simulink model "amplifierboard"  (R2020b)
settings: Solver=FixedStepDiscrete  StartTime=0.0  StopTime=2  FixedStep=0.01  RelTol=1e-3
InitFcn:
  | mbd_s32k_consistency_checks(bdroot(gcs));
undefined symbols (not defined in the file): AutoLowerVal, AutoRaiseVal, HoldVal, LED_En, LED_Off, LED_On, Logic_High, Logic_Low, LQFP, ManualLowerVal, ManualRaiseVal, PWRWNDW_CHDLCK, sC_bool_PWMEN, sC_cnt_FWSetting, sC_cnt_Mtr_DrvNo_HB, sC_cnt_PWMHB1to4, sC_cnt_PWMHB5to8, sC_cnt_TargetSlowRange, sC_pct_ManualMax, sC_pct_RampDwn, sC_pct_RampUp, sC_pct_StartPWM, sC_pct_Targetmax, SwitchPackRangeOffset, Threshold_Value, Tolerant_Time
libraries: mbd_s32k1xx_ec_toolbox x205, simulink x59, canmsglib x19, Filter x15, wndwcmd x3
(part 4 of 6)

== system amplifierboard/CAN_Receive_And_Unpack/Subsystem/Chart/SendPos31StopPosResp ==
  f : TriggerPort  TriggerType=function-call  VariantControl=(inherit)
      settings: CopyFcn=Stateflow.SLINSF.SimulinkMan.removeBlockPreDeleteFcn  PreDeleteFcn=Stateflow.SLINSF.SimulinkMan.unsafePredeleteFcn
  FCAN_Send_ID_0xAA : mbd_s32k1xx_ec_toolbox/Communication Blocks/CAN Blocks/FCAN_Send  Priority=2  can_instance=1  can_mode=Non-blocking  can_timeout_ms=0  can_mb_idx=29  can_mb_init=On each call  show_id_input=off  can_extended_id=off  can_is_remote=off  can_id=AA  show_adv_opts=on  can_fd_enable=off  can_enable_brs=on  can_fd_padding=0
  Generate_Data : Subsystem
  wires:
  Generate_Data/2(Length) -> FCAN_Send_ID_0xAA/2
  Generate_Data/1(Data) -> FCAN_Send_ID_0xAA/1

== system amplifierboard/CAN_Receive_And_Unpack/Subsystem/If Action Subsystem1 ==
  TImeStamp : Inport
  Action Port : ActionPort  ActionPortLabel=if((u1 ~= u2) | ( u3 == 1))
  Constant : Constant  OutDataTypeStr=boolean
  Data Store Write : DataStoreWrite  DataStoreName=PreviousTimeStamp
  Data Store Write1 : DataStoreWrite  DataStoreName=NewMsgRXed
  wires:
  TImeStamp/1 -> Data Store Write/1
  Constant/1 -> Data Store Write1/1

== system amplifierboard/CAN_Receive_And_Unpack/Subsystem/If Action Subsystem2 ==
  Action Port : ActionPort  ActionPortLabel=else
  Constant : Constant  Value=0  OutDataTypeStr=boolean
  Data Store Write1 : DataStoreWrite  DataStoreName=NewMsgRXed
  wires:
  Constant/1 -> Data Store Write1/1

== system amplifierboard/CAN_Receive_And_Unpack/Subsystem1/Fold_Unfold ==
  Input : Inport
  Input1 : Inport  Port=2
  Compare To Constant : simulink/Logic and Bit Operations/Compare To Constant  relop===  const=1.0  OutDataTypeStr=boolean
  Compare To Constant{1..2,4..5} (4 alike) : simulink/Logic and Bit Operations/Compare To Constant  relop===  const=0  OutDataTypeStr=boolean
  Compare To Constant3 : simulink/Logic and Bit Operations/Compare To Constant  relop===  const=1  OutDataTypeStr=boolean
  Compare To Constant6 : simulink/Logic and Bit Operations/Compare To Constant  relop===  const=1  OutDataTypeStr=boolean
  Compare To Constant7 : simulink/Logic and Bit Operations/Compare To Constant  relop===  const=1  OutDataTypeStr=boolean
  If : If  NumInputs=4  IfExpression=u1 == 1  ElseIfExpressions=u2 == 1, u3 == 1 , u4 == 1  ShowElse=off
  If Action Subsystem : Subsystem  TreatAsAtomicUnit=on
  If Action Subsystem1 : Subsystem  TreatAsAtomicUnit=on
  If Action Subsystem2 : Subsystem  TreatAsAtomicUnit=on
  If Action Subsystem3 : Subsystem  TreatAsAtomicUnit=on
  Logical Operator{,1..3} (4 alike) : Logic  AllPortsSameDT=off  OutDataTypeStr=boolean
  Merge : Merge  Inputs=4
  Motor : Outport
  wires:
  Input1/1 -> Compare To Constant7/1, Compare To Constant5/1, Compare To Constant3/1, Compare To Constant1/1
  Compare To Constant5/1 -> Logical Operator2/2
  If Action Subsystem/1("Forward_Direction ") -> Merge/1
  If/2 -> If Action Subsystem1/Action
  Compare To Constant2/1 -> Logical Operator1/1
  Compare To Constant4/1 -> Logical Operator2/1
  Compare To Constant3/1 -> Logical Operator1/2
  Compare To Constant/1 -> Logical Operator/1
  Logical Operator3/1 -> If/4
  Input/1 -> Compare To Constant2/1, Compare To Constant4/1, Compare To Constant6/1, Compare To Constant/1
  Compare To Constant7/1 -> Logical Operator3/2
  If/4 -> If Action Subsystem3/Action
  Compare To Constant6/1 -> Logical Operator3/1
  Merge/1 -> Motor/1
  If Action Subsystem1/1(Reverse_Direction) -> Merge/2
  If Action Subsystem3/1(Standstill_invalid) -> Merge/4
  If Action Subsystem2/1(Standstill_Invalid) -> Merge/3
  If/1 -> If Action Subsystem/Action
  Logical Operator2/1 -> If/3
  Logical Operator1/1 -> If/2
  Compare To Constant1/1 -> Logical Operator/2
  If/3 -> If Action Subsystem2/Action
  Logical Operator/1 -> If/1

== system amplifierboard/CAN_Receive_And_Unpack/Subsystem1/LED1DR_PWM ==
  In1 : Inport
  Data Type Conversion1 : DataTypeConversion  OutDataTypeStr=Enum: LED_En
  Data Type Conversion11 : DataTypeConversion  OutDataTypeStr=Enum: LED_En
  Digital_Output : mbd_s32k1xx_ec_toolbox/GPIO Blocks/Digital_Output  gpio_pin=PTD8: [PTD8 | Port D I/O]  init_val=Low  drive_strength=High
  Enumerated Constant1 : simulink/Sources/Enumerated Constant  OutDataTypeStr=Enum: LED_En  Value=LED_En.DISABLE  SampleTime=inf
  Enumerated Constant6 : simulink/Sources/Enumerated Constant  OutDataTypeStr=Enum: LED_En  Value=LED_En.ENABLE  SampleTime=inf
  LED_Off : Constant  Value=LED_Off  OutDataTypeStr=Inherit: Inherit via back propagation
  LED_On : Constant  Value=LED_On  OutDataTypeStr=Inherit: Inherit via back propagation
  Relational Operator1 : RelationalOperator  Operator===  OutDataTypeStr=boolean  RndMeth=Simplest
  Relational Operator6 : RelationalOperator  Operator===  OutDataTypeStr=boolean  RndMeth=Simplest
  Switch : Switch  Criteria=u2 > Threshold
  Switch1 : Switch  Criteria=u2 > Threshold
  Unit Delay : UnitDelay  SampleTime=-1  HasFrameUpgradeWarning=on
  wires:
  In1/1 -> Data Type Conversion11/1, Data Type Conversion1/1
  Switch1/1 -> Switch/3
  LED_Off/1 -> Switch1/1
  Enumerated Constant6/1 -> Relational Operator6/2
  Data Type Conversion11/1 -> Relational Operator6/1
  Relational Operator1/1 -> Switch1/2
  Relational Operator6/1 -> Switch/2
  LED_On/1 -> Switch/1
  Switch/1 -> Unit Delay/1, Digital_Output/1
  Enumerated Constant1/1 -> Relational Operator1/2
  Data Type Conversion1/1 -> Relational Operator1/1
  Unit Delay/1 -> Switch1/3

== system amplifierboard/CAN_Receive_And_Unpack/Subsystem1/LED2DR_PWM ==
  In1 : Inport
  Data Type Conversion1 : DataTypeConversion  OutDataTypeStr=Enum: LED_En
  Data Type Conversion11 : DataTypeConversion  OutDataTypeStr=Enum: LED_En
  Digital_Output : mbd_s32k1xx_ec_toolbox/GPIO Blocks/Digital_Output  gpio_pin=PTD9: [PTD9 | Port D I/O]  init_val=Low  drive_strength=High
  Enumerated Constant1 : simulink/Sources/Enumerated Constant  OutDataTypeStr=Enum: LED_En  Value=LED_En.DISABLE  SampleTime=inf
  Enumerated Constant6 : simulink/Sources/Enumerated Constant  OutDataTypeStr=Enum: LED_En  Value=LED_En.ENABLE  SampleTime=inf
  LED_Off : Constant  Value=LED_Off  OutDataTypeStr=Inherit: Inherit via back propagation
  LED_On : Constant  Value=LED_On  OutDataTypeStr=Inherit: Inherit via back propagation
  Relational Operator1 : RelationalOperator  Operator===  OutDataTypeStr=boolean  RndMeth=Simplest
  Relational Operator6 : RelationalOperator  Operator===  OutDataTypeStr=boolean  RndMeth=Simplest
  Switch : Switch  Criteria=u2 > Threshold
  Switch1 : Switch  Criteria=u2 > Threshold
  Unit Delay : UnitDelay  SampleTime=-1  HasFrameUpgradeWarning=on
  wires:
  Unit Delay/1 -> Switch1/3
  Data Type Conversion1/1 -> Relational Operator1/1
  Enumerated Constant1/1 -> Relational Operator1/2
  Switch/1 -> Digital_Output/1, Unit Delay/1
  LED_On/1 -> Switch/1
  Relational Operator6/1 -> Switch/2
  Relational Operator1/1 -> Switch1/2
  Data Type Conversion11/1 -> Relational Operator6/1
  Enumerated Constant6/1 -> Relational Operator6/2
  LED_Off/1 -> Switch1/1
  Switch1/1 -> Switch/3
  In1/1 -> Data Type Conversion1/1, Data Type Conversion11/1

== system amplifierboard/CAN_Receive_And_Unpack/Subsystem1/LED3DR_PWM ==
  In1 : Inport
  Data Type Conversion1 : DataTypeConversion  OutDataTypeStr=Enum: LED_En
  Data Type Conversion11 : DataTypeConversion  OutDataTypeStr=Enum: LED_En
  Digital_Output : mbd_s32k1xx_ec_toolbox/GPIO Blocks/Digital_Output  gpio_pin=PTC13: [PTC13 | Port C I/O]  init_val=Low  drive_strength=High
  Enumerated Constant1 : simulink/Sources/Enumerated Constant  OutDataTypeStr=Enum: LED_En  Value=LED_En.DISABLE  SampleTime=inf
  Enumerated Constant6 : simulink/Sources/Enumerated Constant  OutDataTypeStr=Enum: LED_En  Value=LED_En.ENABLE  SampleTime=inf
  LED_Off : Constant  Value=LED_Off  OutDataTypeStr=Inherit: Inherit via back propagation
  LED_On : Constant  Value=LED_On  OutDataTypeStr=Inherit: Inherit via back propagation
  Relational Operator1 : RelationalOperator  Operator===  OutDataTypeStr=boolean  RndMeth=Simplest
  Relational Operator6 : RelationalOperator  Operator===  OutDataTypeStr=boolean  RndMeth=Simplest
  Switch : Switch  Criteria=u2 > Threshold
  Switch1 : Switch  Criteria=u2 > Threshold
  Unit Delay : UnitDelay  SampleTime=-1  HasFrameUpgradeWarning=on
  wires:
  In1/1 -> Data Type Conversion11/1, Data Type Conversion1/1
  Switch1/1 -> Switch/3
  LED_Off/1 -> Switch1/1
  Enumerated Constant6/1 -> Relational Operator6/2
  Data Type Conversion11/1 -> Relational Operator6/1
  Relational Operator1/1 -> Switch1/2
  Relational Operator6/1 -> Switch/2
  LED_On/1 -> Switch/1
  Switch/1 -> Unit Delay/1, Digital_Output/1
  Enumerated Constant1/1 -> Relational Operator1/2
  Data Type Conversion1/1 -> Relational Operator1/1
  Unit Delay/1 -> Switch1/3

== system amplifierboard/CAN_Receive_And_Unpack/Subsystem1/LED4DR_PWM ==
  In1 : Inport
  Data Type Conversion1 : DataTypeConversion  OutDataTypeStr=Enum: LED_En
  Data Type Conversion11 : DataTypeConversion  OutDataTypeStr=Enum: LED_En
  Digital_Output : mbd_s32k1xx_ec_toolbox/GPIO Blocks/Digital_Output  gpio_pin=PTC10: [PTC10 | Port C I/O]  init_val=Low  drive_strength=High
  Enumerated Constant1 : simulink/Sources/Enumerated Constant  OutDataTypeStr=Enum: LED_En  Value=LED_En.DISABLE  SampleTime=inf
  Enumerated Constant6 : simulink/Sources/Enumerated Constant  OutDataTypeStr=Enum: LED_En  Value=LED_En.ENABLE  SampleTime=inf
  LED_Off : Constant  Value=LED_Off  OutDataTypeStr=Inherit: Inherit via back propagation
  LED_On : Constant  Value=LED_On  OutDataTypeStr=Inherit: Inherit via back propagation
  Relational Operator1 : RelationalOperator  Operator===  OutDataTypeStr=boolean  RndMeth=Simplest
  Relational Operator6 : RelationalOperator  Operator===  OutDataTypeStr=boolean  RndMeth=Simplest
  Switch : Switch  Criteria=u2 > Threshold
  Switch1 : Switch  Criteria=u2 > Threshold
  Unit Delay : UnitDelay  SampleTime=-1  HasFrameUpgradeWarning=on
  wires:
  Unit Delay/1 -> Switch1/3
  Data Type Conversion1/1 -> Relational Operator1/1
  Enumerated Constant1/1 -> Relational Operator1/2
  Switch/1 -> Digital_Output/1, Unit Delay/1
  LED_On/1 -> Switch/1
  Relational Operator6/1 -> Switch/2
  Relational Operator1/1 -> Switch1/2
  Data Type Conversion11/1 -> Relational Operator6/1
  Enumerated Constant6/1 -> Relational Operator6/2
  LED_Off/1 -> Switch1/1
  Switch1/1 -> Switch/3
  In1/1 -> Data Type Conversion1/1, Data Type Conversion11/1

== system amplifierboard/CAN_Receive_And_Unpack/Subsystem1/LED5DR_PWM ==
  In1 : Inport
  Data Type Conversion1 : DataTypeConversion  OutDataTypeStr=Enum: LED_En
  Data Type Conversion11 : DataTypeConversion  OutDataTypeStr=Enum: LED_En
  Digital_Output : mbd_s32k1xx_ec_toolbox/GPIO Blocks/Digital_Output  gpio_pin=PTC11: [PTC11 | Port C I/O]  init_val=Low  drive_strength=High
  Enumerated Constant1 : simulink/Sources/Enumerated Constant  OutDataTypeStr=Enum: LED_En  Value=LED_En.DISABLE  SampleTime=inf
  Enumerated Constant6 : simulink/Sources/Enumerated Constant  OutDataTypeStr=Enum: LED_En  Value=LED_En.ENABLE  SampleTime=inf
  LED_Off : Constant  Value=LED_Off  OutDataTypeStr=Inherit: Inherit via back propagation
  LED_On : Constant  Value=LED_On  OutDataTypeStr=Inherit: Inherit via back propagation
  Relational Operator1 : RelationalOperator  Operator===  OutDataTypeStr=boolean  RndMeth=Simplest
  Relational Operator6 : RelationalOperator  Operator===  OutDataTypeStr=boolean  RndMeth=Simplest
  Switch : Switch  Criteria=u2 > Threshold
  Switch1 : Switch  Criteria=u2 > Threshold
  Unit Delay : UnitDelay  SampleTime=-1  HasFrameUpgradeWarning=on
  wires:
  In1/1 -> Data Type Conversion11/1, Data Type Conversion1/1
  Switch1/1 -> Switch/3
  LED_Off/1 -> Switch1/1
  Enumerated Constant6/1 -> Relational Operator6/2
  Data Type Conversion11/1 -> Relational Operator6/1
  Relational Operator1/1 -> Switch1/2
  Relational Operator6/1 -> Switch/2
  LED_On/1 -> Switch/1
  Switch/1 -> Unit Delay/1, Digital_Output/1
  Enumerated Constant1/1 -> Relational Operator1/2
  Data Type Conversion1/1 -> Relational Operator1/1
  Unit Delay/1 -> Switch1/3

== system amplifierboard/CAN_Receive_And_Unpack/Subsystem1/LED6DR_PWM ==
  In1 : Inport
  Data Type Conversion1 : DataTypeConversion  OutDataTypeStr=Enum: LED_En
  Data Type Conversion11 : DataTypeConversion  OutDataTypeStr=Enum: LED_En
  Digital_Output : mbd_s32k1xx_ec_toolbox/GPIO Blocks/Digital_Output  gpio_pin=PTC9: [PTC9 | Port C I/O]  init_val=Low  drive_strength=High
  Enumerated Constant1 : simulink/Sources/Enumerated Constant  OutDataTypeStr=Enum: LED_En  Value=LED_En.DISABLE  SampleTime=inf
  Enumerated Constant6 : simulink/Sources/Enumerated Constant  OutDataTypeStr=Enum: LED_En  Value=LED_En.ENABLE  SampleTime=inf
  LED_Off : Constant  Value=LED_Off  OutDataTypeStr=Inherit: Inherit via back propagation
  LED_On : Constant  Value=LED_On  OutDataTypeStr=Inherit: Inherit via back propagation
  Relational Operator1 : RelationalOperator  Operator===  OutDataTypeStr=boolean  RndMeth=Simplest
  Relational Operator6 : RelationalOperator  Operator===  OutDataTypeStr=boolean  RndMeth=Simplest
  Switch : Switch  Criteria=u2 > Threshold
  Switch1 : Switch  Criteria=u2 > Threshold
  Unit Delay : UnitDelay  SampleTime=-1  HasFrameUpgradeWarning=on
  wires:
  Unit Delay/1 -> Switch1/3
  Data Type Conversion1/1 -> Relational Operator1/1
  Enumerated Constant1/1 -> Relational Operator1/2
  Switch/1 -> Digital_Output/1, Unit Delay/1
  LED_On/1 -> Switch/1
  Relational Operator6/1 -> Switch/2
  Relational Operator1/1 -> Switch1/2
  Data Type Conversion11/1 -> Relational Operator6/1
  Enumerated Constant6/1 -> Relational Operator6/2
  LED_Off/1 -> Switch1/1
  Switch1/1 -> Switch/3
  In1/1 -> Data Type Conversion1/1, Data Type Conversion11/1

== system amplifierboard/CAN_Receive_And_Unpack/Subsystem1/Motor4 ==
  Input : Inport
  Input1 : Inport  Port=2
  Compare To Constant : simulink/Logic and Bit Operations/Compare To Constant  relop===  const=1.0  OutDataTypeStr=boolean
  Compare To Constant{1..2,4..5} (4 alike) : simulink/Logic and Bit Operations/Compare To Constant  relop===  const=0  OutDataTypeStr=boolean
  Compare To Constant3 : simulink/Logic and Bit Operations/Compare To Constant  relop===  const=1  OutDataTypeStr=boolean
  Compare To Constant6 : simulink/Logic and Bit Operations/Compare To Constant  relop===  const=1  OutDataTypeStr=boolean
  Compare To Constant7 : simulink/Logic and Bit Operations/Compare To Constant  relop===  const=1  OutDataTypeStr=boolean
  If : If  NumInputs=4  IfExpression=u1 == 1  ElseIfExpressions=u2 == 1, u3 == 1 , u4 == 1  ShowElse=off
  If Action Subsystem : Subsystem  TreatAsAtomicUnit=on
  If Action Subsystem1 : Subsystem  TreatAsAtomicUnit=on
  If Action Subsystem2 : Subsystem  TreatAsAtomicUnit=on
  If Action Subsystem3 : Subsystem  TreatAsAtomicUnit=on
  Logical Operator{,1..3} (4 alike) : Logic  AllPortsSameDT=off  OutDataTypeStr=boolean
  Merge : Merge  Inputs=4
  Motor : Outport
  wires:
  Logical Operator/1 -> If/1
  If/3 -> If Action Subsystem2/Action
  Compare To Constant1/1 -> Logical Operator/2
  Logical Operator1/1 -> If/2
  Logical Operator2/1 -> If/3
  If/1 -> If Action Subsystem/Action
  If Action Subsystem2/1(Standstill_Invalid) -> Merge/3
  If Action Subsystem3/1(Standstill_invalid) -> Merge/4
  If Action Subsystem1/1(Reverse_Direction) -> Merge/2
  Merge/1 -> Motor/1
  Compare To Constant6/1 -> Logical Operator3/1
  If/4 -> If Action Subsystem3/Action
  Compare To Constant7/1 -> Logical Operator3/2
  Input/1 -> Compare To Constant/1, Compare To Constant6/1, Compare To Constant4/1, Compare To Constant2/1
  Logical Operator3/1 -> If/4
  Compare To Constant/1 -> Logical Operator/1
  Compare To Constant3/1 -> Logical Operator1/2
  Compare To Constant4/1 -> Logical Operator2/1
  Compare To Constant2/1 -> Logical Operator1/1
  If/2 -> If Action Subsystem1/Action
  If Action Subsystem/1("Forward_Direction ") -> Merge/1
  Compare To Constant5/1 -> Logical Operator2/2
  Input1/1 -> Compare To Constant1/1, Compare To Constant3/1, Compare To Constant5/1, Compare To Constant7/1

== system amplifierboard/CAN_Receive_And_Unpack/Subsystem1/Motor5 ==
  Input : Inport
  Heating : Inport  Port=2
  Compare To Constant : simulink/Logic and Bit Operations/Compare To Constant  relop===  const=1.0  OutDataTypeStr=boolean
  Compare To Constant1 : simulink/Logic and Bit Operations/Compare To Constant  relop===  const=0  OutDataTypeStr=boolean
  Compare To Constant2 : simulink/Logic and Bit Operations/Compare To Constant  relop===  const=0  OutDataTypeStr=boolean
  Compare To Constant3 : simulink/Logic and Bit Operations/Compare To Constant  relop===  const=1  OutDataTypeStr=boolean
  If : If  NumInputs=2  IfExpression=u2 == 1
  If Action Subsystem : Subsystem  TreatAsAtomicUnit=on
  If Action Subsystem1 : Subsystem  TreatAsAtomicUnit=on
  Logical Operator : Logic  AllPortsSameDT=off  OutDataTypeStr=boolean
  Logical Operator1 : Logic  AllPortsSameDT=off  OutDataTypeStr=boolean
  Merge : Merge
  Motor : Outport
  wires:
  Heating/1 -> Compare To Constant1/1, Compare To Constant3/1
  If Action Subsystem/1("Forward_Direction ") -> Merge/1
  If/2 -> If Action Subsystem1/Action
  Compare To Constant2/1 -> Logical Operator1/1
  Compare To Constant3/1 -> Logical Operator1/2
  Compare To Constant/1 -> Logical Operator/1
  Input/1 -> Compare To Constant2/1, Compare To Constant/1
  Merge/1 -> Motor/1
  If Action Subsystem1/1(Standstill_Invalid) -> Merge/2
  If/1 -> If Action Subsystem/Action
  Logical Operator1/1 -> If/2
  Compare To Constant1/1 -> Logical Operator/2
  Logical Operator/1 -> If/1

== system amplifierboard/CAN_Receive_And_Unpack/Subsystem1/Motor6 ==
  Input : Inport
  Input1 : Inport  Port=2
  Compare To Constant : simulink/Logic and Bit Operations/Compare To Constant  relop===  const=1.0  OutDataTypeStr=boolean
  Compare To Constant{1..2,4..5} (4 alike) : simulink/Logic and Bit Operations/Compare To Constant  relop===  const=0  OutDataTypeStr=boolean
  Compare To Constant3 : simulink/Logic and Bit Operations/Compare To Constant  relop===  const=1  OutDataTypeStr=boolean
  Compare To Constant6 : simulink/Logic and Bit Operations/Compare To Constant  relop===  const=1  OutDataTypeStr=boolean
  Compare To Constant7 : simulink/Logic and Bit Operations/Compare To Constant  relop===  const=1  OutDataTypeStr=boolean
  If : If  NumInputs=4  IfExpression=u1 == 1  ElseIfExpressions=u2 == 1, u3 == 1 , u4 == 1  ShowElse=off
  If Action Subsystem : Subsystem  TreatAsAtomicUnit=on
  If Action Subsystem1 : Subsystem  TreatAsAtomicUnit=on
  If Action Subsystem2 : Subsystem  TreatAsAtomicUnit=on
  If Action Subsystem3 : Subsystem  TreatAsAtomicUnit=on
  Logical Operator{,1..3} (4 alike) : Logic  AllPortsSameDT=off  OutDataTypeStr=boolean
  Merge : Merge  Inputs=4
  Motor : Outport
  wires:
  Logical Operator/1 -> If/1
  If/3 -> If Action Subsystem2/Action
  Compare To Constant1/1 -> Logical Operator/2
  Logical Operator1/1 -> If/2
  Logical Operator2/1 -> If/3
  If/1 -> If Action Subsystem/Action
  If Action Subsystem2/1(Standstill_Invalid) -> Merge/3
  If Action Subsystem3/1(Standstill_invalid) -> Merge/4
  If Action Subsystem1/1(Reverse_Direction) -> Merge/2
  Merge/1 -> Motor/1
  Compare To Constant6/1 -> Logical Operator3/1
  If/4 -> If Action Subsystem3/Action
  Compare To Constant7/1 -> Logical Operator3/2
  Input/1 -> Compare To Constant/1, Compare To Constant6/1, Compare To Constant4/1, Compare To Constant2/1
  Logical Operator3/1 -> If/4
  Compare To Constant/1 -> Logical Operator/1
  Compare To Constant3/1 -> Logical Operator1/2
  Compare To Constant4/1 -> Logical Operator2/1
  Compare To Constant2/1 -> Logical Operator1/1
  If/2 -> If Action Subsystem1/Action
  If Action Subsystem/1("Forward_Direction ") -> Merge/1
  Compare To Constant5/1 -> Logical Operator2/2
  Input1/1 -> Compare To Constant1/1, Compare To Constant3/1, Compare To Constant5/1, Compare To Constant7/1

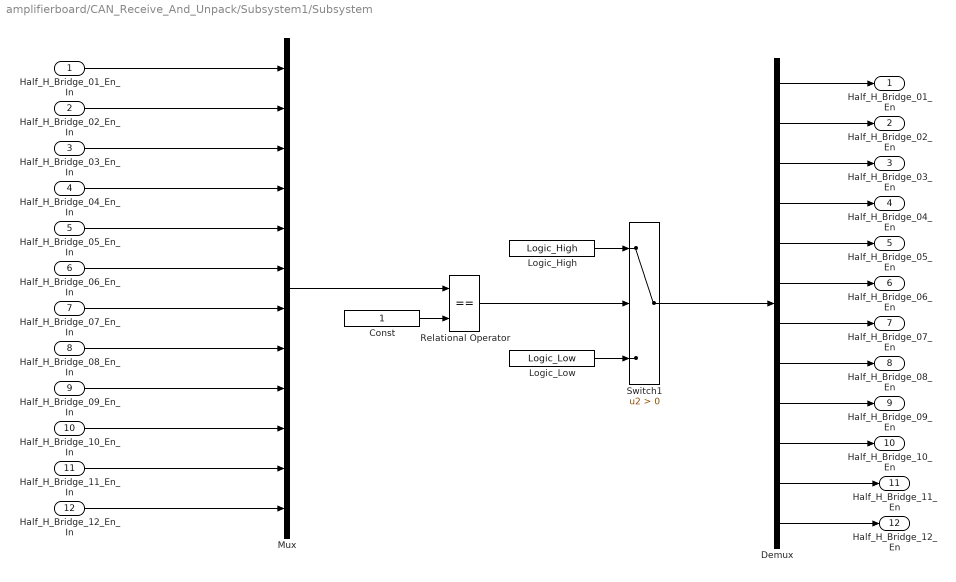
== system amplifierboard/CAN_Receive_And_Unpack/Subsystem1/Subsystem ==
  Half_H_Bridge_01_En_In : Inport
  Half_H_Bridge_02_En_In : Inport  Port=2
  Half_H_Bridge_03_En_In : Inport  Port=3
  Half_H_Bridge_04_En_In : Inport  Port=4
  Half_H_Bridge_05_En_In : Inport  Port=5
  Half_H_Bridge_06_En_In : Inport  Port=6
  Half_H_Bridge_07_En_In : Inport  Port=7
  Half_H_Bridge_08_En_In : Inport  Port=8
  Half_H_Bridge_09_En_In : Inport  Port=9
  Half_H_Bridge_10_En_In : Inport  Port=10
  Half_H_Bridge_11_En_In : Inport  Port=11
  Half_H_Bridge_12_En_In : Inport  Port=12
  Const : Constant  OutDataTypeStr=Inherit: Inherit via back propagation
  Demux : Demux  Outputs=12
  Logic_High : Constant  Value=Logic_High  OutDataTypeStr=Inherit: Inherit via back propagation
  Logic_Low : Constant  Value=Logic_Low  OutDataTypeStr=Inherit: Inherit via back propagation
  Mux : Mux  Inputs=12
  Relational Operator : RelationalOperator  Operator===  OutDataTypeStr=boolean  RndMeth=Simplest
  Switch1 : Switch  Criteria=u2 > Threshold
  Half_H_Bridge_01_En : Outport
  Half_H_Bridge_02_En : Outport  Port=2
  Half_H_Bridge_03_En : Outport  Port=3
  Half_H_Bridge_04_En : Outport  Port=4
  Half_H_Bridge_05_En : Outport  Port=5
  Half_H_Bridge_06_En : Outport  Port=6
  Half_H_Bridge_07_En : Outport  Port=7
  Half_H_Bridge_08_En : Outport  Port=8
  Half_H_Bridge_09_En : Outport  Port=9
  Half_H_Bridge_10_En : Outport  Port=10
  Half_H_Bridge_11_En : Outport  Port=11
  Half_H_Bridge_12_En : Outport  Port=12
  wires:
  Relational Operator/1 -> Switch1/2
  Switch1/1 -> Demux/1
  Demux/1 -> Half_H_Bridge_01_En/1
  Half_H_Bridge_02_En_In/1 -> Mux/2
  Half_H_Bridge_03_En_In/1 -> Mux/3
  Half_H_Bridge_04_En_In/1 -> Mux/4
  Half_H_Bridge_05_En_In/1 -> Mux/5
  Demux/2 -> Half_H_Bridge_02_En/1
  Demux/3 -> Half_H_Bridge_03_En/1
  Demux/4 -> Half_H_Bridge_04_En/1
  Demux/5 -> Half_H_Bridge_05_En/1
  Half_H_Bridge_06_En_In/1 -> Mux/6
  Half_H_Bridge_07_En_In/1 -> Mux/7
  Half_H_Bridge_08_En_In/1 -> Mux/8
  Half_H_Bridge_09_En_In/1 -> Mux/9
  Half_H_Bridge_10_En_In/1 -> Mux/10
  Half_H_Bridge_11_En_In/1 -> Mux/11
  Half_H_Bridge_12_En_In/1 -> Mux/12
  Demux/6 -> Half_H_Bridge_06_En/1
  Demux/7 -> Half_H_Bridge_07_En/1
  Demux/8 -> Half_H_Bridge_08_En/1
  Demux/9 -> Half_H_Bridge_09_En/1
  Demux/10 -> Half_H_Bridge_10_En/1
  Demux/11 -> Half_H_Bridge_11_En/1
  Demux/12 -> Half_H_Bridge_12_En/1
  Half_H_Bridge_01_En_In/1 -> Mux/1
  Mux/1 -> Relational Operator/1
  Const/1 -> Relational Operator/2
  Logic_Low/1 -> Switch1/3
  Logic_High/1 -> Switch1/1

== system amplifierboard/CAN_Receive_And_Unpack/Subsystem1/Subsystem1 ==
  mirror_common : Inport
  right_left : Inport  Port=2
  up_down : Inport  Port=3
  Motor2 : Subsystem
  Motor3 : Subsystem
  Motor4 : Outport
  Motor5 : Outport  Port=2
  wires:
  Motor2/1(Motor) -> Motor4/1
  Motor3/1(Motor) -> Motor5/1
  up_down/1 -> Motor3/1(Input)
  right_left/1 -> Motor2/1(Input)
  mirror_common/1 -> Motor3/2(Input1), Motor2/2(Input1)

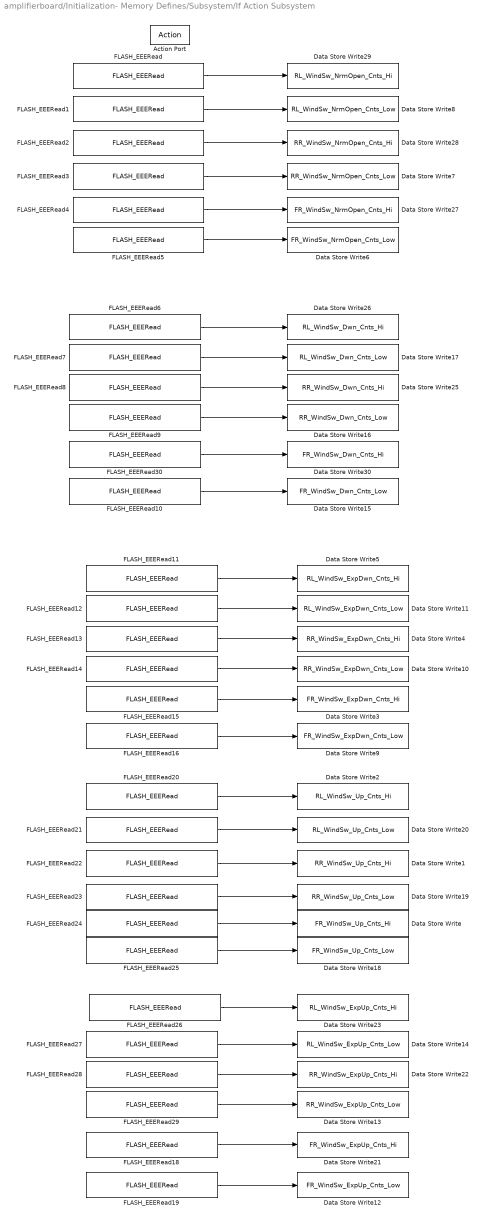
== system amplifierboard/Initialization- Memory Defines/Subsystem/If Action Subsystem ==
  Action Port : ActionPort  ActionPortLabel=if((u1 <= 1200) & (u2 <= 750))
  Data Store Write : DataStoreWrite  DataStoreName=FR_WindSw_Up_Cnts_Hi
  Data Store Write1 : DataStoreWrite  DataStoreName=RR_WindSw_Up_Cnts_Hi
  Data Store Write10 : DataStoreWrite  DataStoreName=RR_WindSw_ExpDwn_Cnts_Low
  Data Store Write11 : DataStoreWrite  DataStoreName=RL_WindSw_ExpDwn_Cnts_Low
  Data Store Write12 : DataStoreWrite  DataStoreName=FR_WindSw_ExpUp_Cnts_Low
  Data Store Write13 : DataStoreWrite  DataStoreName=RR_WindSw_ExpUp_Cnts_Low
  Data Store Write14 : DataStoreWrite  DataStoreName=RL_WindSw_ExpUp_Cnts_Low
  Data Store Write15 : DataStoreWrite  DataStoreName=FR_WindSw_Dwn_Cnts_Low
  Data Store Write16 : DataStoreWrite  DataStoreName=RR_WindSw_Dwn_Cnts_Low
  Data Store Write17 : DataStoreWrite  DataStoreName=RL_WindSw_Dwn_Cnts_Low
  Data Store Write18 : DataStoreWrite  DataStoreName=FR_WindSw_Up_Cnts_Low
  Data Store Write19 : DataStoreWrite  DataStoreName=RR_WindSw_Up_Cnts_Low
  Data Store Write2 : DataStoreWrite  DataStoreName=RL_WindSw_Up_Cnts_Hi
  Data Store Write20 : DataStoreWrite  DataStoreName=RL_WindSw_Up_Cnts_Low
  Data Store Write21 : DataStoreWrite  DataStoreName=FR_WindSw_ExpUp_Cnts_Hi
  Data Store Write22 : DataStoreWrite  DataStoreName=RR_WindSw_ExpUp_Cnts_Hi
  Data Store Write23 : DataStoreWrite  DataStoreName=RL_WindSw_ExpUp_Cnts_Hi
  Data Store Write25 : DataStoreWrite  DataStoreName=RR_WindSw_Dwn_Cnts_Hi
  Data Store Write26 : DataStoreWrite  DataStoreName=RL_WindSw_Dwn_Cnts_Hi
  Data Store Write27 : DataStoreWrite  DataStoreName=FR_WindSw_NrmOpen_Cnts_Hi
  Data Store Write28 : DataStoreWrite  DataStoreName=RR_WindSw_NrmOpen_Cnts_Hi
  Data Store Write29 : DataStoreWrite  DataStoreName=RL_WindSw_NrmOpen_Cnts_Hi
  Data Store Write3 : DataStoreWrite  DataStoreName=FR_WindSw_ExpDwn_Cnts_Hi
  Data Store Write30 : DataStoreWrite  DataStoreName=FR_WindSw_Dwn_Cnts_Hi
  Data Store Write4 : DataStoreWrite  DataStoreName=RR_WindSw_ExpDwn_Cnts_Hi
  Data Store Write5 : DataStoreWrite  DataStoreName=RL_WindSw_ExpDwn_Cnts_Hi
  Data Store Write6 : DataStoreWrite  DataStoreName=FR_WindSw_NrmOpen_Cnts_Low
  Data Store Write7 : DataStoreWrite  DataStoreName=RR_WindSw_NrmOpen_Cnts_Low
  Data Store Write8 : DataStoreWrite  DataStoreName=RL_WindSw_NrmOpen_Cnts_Low
  Data Store Write9 : DataStoreWrite  DataStoreName=FR_WindSw_ExpDwn_Cnts_Low
  FLASH_EEERead : mbd_s32k1xx_ec_toolbox/Core and System Blocks/FLASH Blocks/FLASH_EEERead  base=0x14000000  offset=0x0F00  ptr=uint16_t
  FLASH_EEERead1 : mbd_s32k1xx_ec_toolbox/Core and System Blocks/FLASH Blocks/FLASH_EEERead  base=0x14000000  offset=0x0F02  ptr=uint16_t
  FLASH_EEERead10 : mbd_s32k1xx_ec_toolbox/Core and System Blocks/FLASH Blocks/FLASH_EEERead  base=0x14000000  offset=0x0F16  ptr=uint16_t
  FLASH_EEERead11 : mbd_s32k1xx_ec_toolbox/Core and System Blocks/FLASH Blocks/FLASH_EEERead  base=0x14000000  offset=0x0F18  ptr=uint16_t
  FLASH_EEERead12 : mbd_s32k1xx_ec_toolbox/Core and System Blocks/FLASH Blocks/FLASH_EEERead  base=0x14000000  offset=0x0F1A  ptr=uint16_t
  FLASH_EEERead13 : mbd_s32k1xx_ec_toolbox/Core and System Blocks/FLASH Blocks/FLASH_EEERead  base=0x14000000  offset=0x0F1C  ptr=uint16_t
  FLASH_EEERead14 : mbd_s32k1xx_ec_toolbox/Core and System Blocks/FLASH Blocks/FLASH_EEERead  base=0x14000000  offset=0x0F1E  ptr=uint16_t
  FLASH_EEERead15 : mbd_s32k1xx_ec_toolbox/Core and System Blocks/FLASH Blocks/FLASH_EEERead  base=0x14000000  offset=0x0F20  ptr=uint16_t
  FLASH_EEERead16 : mbd_s32k1xx_ec_toolbox/Core and System Blocks/FLASH Blocks/FLASH_EEERead  base=0x14000000  offset=0x0F22  ptr=uint16_t
  FLASH_EEERead18 : mbd_s32k1xx_ec_toolbox/Core and System Blocks/FLASH Blocks/FLASH_EEERead  base=0x14000000  offset=0x0F38  ptr=uint16_t
  FLASH_EEERead19 : mbd_s32k1xx_ec_toolbox/Core and System Blocks/FLASH Blocks/FLASH_EEERead  base=0x14000000  offset=0x0F3A  ptr=uint16_t
  FLASH_EEERead2 : mbd_s32k1xx_ec_toolbox/Core and System Blocks/FLASH Blocks/FLASH_EEERead  base=0x14000000  offset=0x0F04  ptr=uint16_t
  FLASH_EEERead20 : mbd_s32k1xx_ec_toolbox/Core and System Blocks/FLASH Blocks/FLASH_EEERead  base=0x14000000  offset=0x0F24  ptr=uint16_t
  FLASH_EEERead21 : mbd_s32k1xx_ec_toolbox/Core and System Blocks/FLASH Blocks/FLASH_EEERead  base=0x14000000  offset=0x0F26  ptr=uint16_t
  FLASH_EEERead22 : mbd_s32k1xx_ec_toolbox/Core and System Blocks/FLASH Blocks/FLASH_EEERead  base=0x14000000  offset=0x0F28  ptr=uint16_t
  FLASH_EEERead23 : mbd_s32k1xx_ec_toolbox/Core and System Blocks/FLASH Blocks/FLASH_EEERead  base=0x14000000  offset=0x0F2A  ptr=uint16_t
  FLASH_EEERead24 : mbd_s32k1xx_ec_toolbox/Core and System Blocks/FLASH Blocks/FLASH_EEERead  base=0x14000000  offset=0x0F2C  ptr=uint16_t
  FLASH_EEERead25 : mbd_s32k1xx_ec_toolbox/Core and System Blocks/FLASH Blocks/FLASH_EEERead  base=0x14000000  offset=0x0F2E  ptr=uint16_t
  FLASH_EEERead26 : mbd_s32k1xx_ec_toolbox/Core and System Blocks/FLASH Blocks/FLASH_EEERead  base=0x14000000  offset=0x0F30  ptr=uint16_t
  FLASH_EEERead27 : mbd_s32k1xx_ec_toolbox/Core and System Blocks/FLASH Blocks/FLASH_EEERead  base=0x14000000  offset=0x0F32  ptr=uint16_t
  FLASH_EEERead28 : mbd_s32k1xx_ec_toolbox/Core and System Blocks/FLASH Blocks/FLASH_EEERead  base=0x14000000  offset=0x0F34  ptr=uint16_t
  FLASH_EEERead29 : mbd_s32k1xx_ec_toolbox/Core and System Blocks/FLASH Blocks/FLASH_EEERead  base=0x14000000  offset=0x0F36  ptr=uint16_t
  FLASH_EEERead3 : mbd_s32k1xx_ec_toolbox/Core and System Blocks/FLASH Blocks/FLASH_EEERead  base=0x14000000  offset=0x0F06  ptr=uint16_t
  FLASH_EEERead30 : mbd_s32k1xx_ec_toolbox/Core and System Blocks/FLASH Blocks/FLASH_EEERead  base=0x14000000  offset=0x0F14  ptr=uint16_t
  FLASH_EEERead4 : mbd_s32k1xx_ec_toolbox/Core and System Blocks/FLASH Blocks/FLASH_EEERead  base=0x14000000  offset=0x0F08  ptr=uint16_t
  FLASH_EEERead5 : mbd_s32k1xx_ec_toolbox/Core and System Blocks/FLASH Blocks/FLASH_EEERead  base=0x14000000  offset=0x0F0A  ptr=uint16_t
  FLASH_EEERead6 : mbd_s32k1xx_ec_toolbox/Core and System Blocks/FLASH Blocks/FLASH_EEERead  base=0x14000000  offset=0x0F0C  ptr=uint16_t
  FLASH_EEERead7 : mbd_s32k1xx_ec_toolbox/Core and System Blocks/FLASH Blocks/FLASH_EEERead  base=0x14000000  offset=0x0F0E  ptr=uint16_t
  FLASH_EEERead8 : mbd_s32k1xx_ec_toolbox/Core and System Blocks/FLASH Blocks/FLASH_EEERead  base=0x14000000  offset=0x0F10  ptr=uint16_t
  FLASH_EEERead9 : mbd_s32k1xx_ec_toolbox/Core and System Blocks/FLASH Blocks/FLASH_EEERead  base=0x14000000  offset=0x0F12  ptr=uint16_t
  wires:
  FLASH_EEERead24/1 -> Data Store Write/1
  FLASH_EEERead21/1 -> Data Store Write20/1
  FLASH_EEERead25/1 -> Data Store Write18/1
  FLASH_EEERead23/1 -> Data Store Write19/1
  FLASH_EEERead22/1 -> Data Store Write1/1
  FLASH_EEERead15/1 -> Data Store Write3/1
  FLASH_EEERead20/1 -> Data Store Write2/1
  FLASH_EEERead5/1 -> Data Store Write6/1
  FLASH_EEERead26/1 -> Data Store Write23/1
  FLASH_EEERead13/1 -> Data Store Write4/1
  FLASH_EEERead10/1 -> Data Store Write15/1
  FLASH_EEERead8/1 -> Data Store Write25/1
  FLASH_EEERead29/1 -> Data Store Write13/1
  FLASH_EEERead27/1 -> Data Store Write14/1
  FLASH_EEERead/1 -> Data Store Write29/1
  FLASH_EEERead12/1 -> Data Store Write11/1
  FLASH_EEERead9/1 -> Data Store Write16/1
  FLASH_EEERead1/1 -> Data Store Write8/1
  FLASH_EEERead4/1 -> Data Store Write27/1
  FLASH_EEERead30/1 -> Data Store Write30/1
  FLASH_EEERead19/1 -> Data Store Write12/1
  FLASH_EEERead28/1 -> Data Store Write22/1
  FLASH_EEERead7/1 -> Data Store Write17/1
  FLASH_EEERead16/1 -> Data Store Write9/1
  FLASH_EEERead3/1 -> Data Store Write7/1
  FLASH_EEERead6/1 -> Data Store Write26/1
  FLASH_EEERead18/1 -> Data Store Write21/1
  FLASH_EEERead2/1 -> Data Store Write28/1
  FLASH_EEERead11/1 -> Data Store Write5/1
  FLASH_EEERead14/1 -> Data Store Write10/1

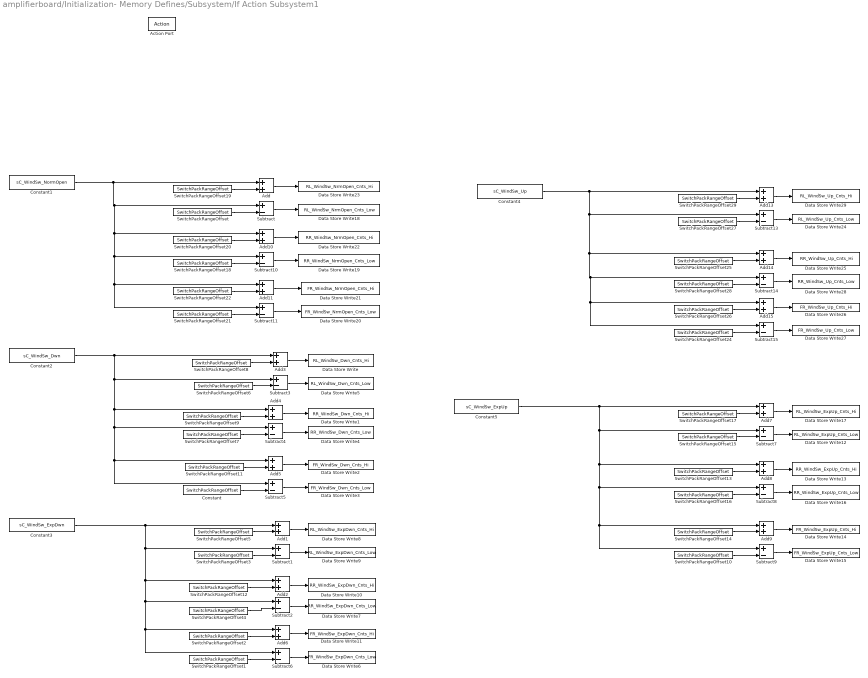
== system amplifierboard/Initialization- Memory Defines/Subsystem/If Action Subsystem1 ==
  Action Port : ActionPort  ActionPortLabel=else
  Add{,1,4..5,7..11,13..15} (12 alike) : Sum
  Add2 : Sum  OutDataTypeStr=uint16
  Add3 : Sum  OutDataTypeStr=uint16
  Add6 : Sum  OutDataTypeStr=uint16
  Constant : Constant  Value=SwitchPackRangeOffset  OutDataTypeStr=uint16
  Constant1 : Constant  Value=sC_WindSw_NormOpen  OutDataTypeStr=uint16
  Constant2 : Constant  Value=sC_WindSw_Dwn  OutDataTypeStr=uint16
  Constant3 : Constant  Value=sC_WindSw_ExpDwn  OutDataTypeStr=uint16
  Constant4 : Constant  Value=sC_WindSw_Up  OutDataTypeStr=uint16
  Constant5 : Constant  Value=sC_WindSw_ExpUp  OutDataTypeStr=uint16
  Data Store Write : DataStoreWrite  DataStoreName=RL_WindSw_Dwn_Cnts_Hi
  Data Store Write1 : DataStoreWrite  DataStoreName=RR_WindSw_Dwn_Cnts_Hi
  Data Store Write10 : DataStoreWrite  DataStoreName=RR_WindSw_ExpDwn_Cnts_Hi
  Data Store Write11 : DataStoreWrite  DataStoreName=FR_WindSw_ExpDwn_Cnts_Hi
  Data Store Write12 : DataStoreWrite  DataStoreName=RL_WindSw_ExpUp_Cnts_Low
  Data Store Write13 : DataStoreWrite  DataStoreName=RR_WindSw_ExpUp_Cnts_Hi
  Data Store Write14 : DataStoreWrite  DataStoreName=FR_WindSw_ExpUp_Cnts_Hi
  Data Store Write15 : DataStoreWrite  DataStoreName=FR_WindSw_ExpUp_Cnts_Low
  Data Store Write16 : DataStoreWrite  DataStoreName=RR_WindSw_ExpUp_Cnts_Low
  Data Store Write17 : DataStoreWrite  DataStoreName=RL_WindSw_ExpUp_Cnts_Hi
  Data Store Write18 : DataStoreWrite  DataStoreName=RL_WindSw_NrmOpen_Cnts_Low
  Data Store Write19 : DataStoreWrite  DataStoreName=RR_WindSw_NrmOpen_Cnts_Low
  Data Store Write2 : DataStoreWrite  DataStoreName=FR_WindSw_Dwn_Cnts_Hi
  Data Store Write20 : DataStoreWrite  DataStoreName=FR_WindSw_NrmOpen_Cnts_Low
  Data Store Write21 : DataStoreWrite  DataStoreName=FR_WindSw_NrmOpen_Cnts_Hi
  Data Store Write22 : DataStoreWrite  DataStoreName=RR_WindSw_NrmOpen_Cnts_Hi
  Data Store Write23 : DataStoreWrite  DataStoreName=RL_WindSw_NrmOpen_Cnts_Hi
  Data Store Write24 : DataStoreWrite  DataStoreName=RL_WindSw_Up_Cnts_Low
  Data Store Write25 : DataStoreWrite  DataStoreName=RR_WindSw_Up_Cnts_Hi
  Data Store Write26 : DataStoreWrite  DataStoreName=FR_WindSw_Up_Cnts_Hi
  Data Store Write27 : DataStoreWrite  DataStoreName=FR_WindSw_Up_Cnts_Low
  Data Store Write28 : DataStoreWrite  DataStoreName=RR_WindSw_Up_Cnts_Low
  Data Store Write29 : DataStoreWrite  DataStoreName=RL_WindSw_Up_Cnts_Hi
  Data Store Write3 : DataStoreWrite  DataStoreName=FR_WindSw_Dwn_Cnts_Low
  Data Store Write4 : DataStoreWrite  DataStoreName=RR_WindSw_Dwn_Cnts_Low
  Data Store Write5 : DataStoreWrite  DataStoreName=RL_WindSw_Dwn_Cnts_Low
  Data Store Write6 : DataStoreWrite  DataStoreName=FR_WindSw_ExpDwn_Cnts_Low
  Data Store Write7 : DataStoreWrite  DataStoreName=RR_WindSw_ExpDwn_Cnts_Low
  Data Store Write8 : DataStoreWrite  DataStoreName=RL_WindSw_ExpDwn_Cnts_Hi
  Data Store Write9 : DataStoreWrite  DataStoreName=RL_WindSw_ExpDwn_Cnts_Low
  Subtract{,1,3..5,7..11,13..15} (13 alike) : Sum  Inputs=+-
  Subtract2 : Sum  Inputs=+-  OutDataTypeStr=uint16
  Subtract6 : Sum  Inputs=+-  OutDataTypeStr=uint16
  SwitchPackRangeOffset{,1..2,6..11,13..22,24..29} (25 alike) : Constant  Value=SwitchPackRangeOffset  OutDataTypeStr=uint16
  SwitchPackRangeOffset{3..5,12} (4 alike) : Constant  Value=SwitchPackRangeOffset  OutDataTypeStr=Inherit: Inherit via back propagation
  wires:
  Subtract2/1 -> Data Store Write7/1
  SwitchPackRangeOffset29/1 -> Add13/2
  Add15/1 -> Data Store Write26/1
  Subtract15/1 -> Data Store Write27/1
  SwitchPackRangeOffset28/1 -> Subtract14/2
  Subtract14/1 -> Data Store Write28/1
  Constant4/1 -> Subtract13/1, Add14/1, Add15/1, Subtract15/1, Subtract14/1, Add13/1
  Add13/1 -> Data Store Write29/1
  Subtract13/1 -> Data Store Write24/1
  SwitchPackRangeOffset26/1 -> Add15/2
  SwitchPackRangeOffset25/1 -> Add14/2
  Constant/1 -> Subtract5/2
  SwitchPackRangeOffset7/1 -> Subtract4/2
  SwitchPackRangeOffset11/1 -> Add5/2
  Add3/1 -> Data Store Write/1
  Add4/1 -> Data Store Write1/1
  Constant2/1 -> Subtract3/1, Add4/1, Subtract4/1, Add5/1, Subtract5/1, Add3/1
  Add14/1 -> Data Store Write25/1
  Add5/1 -> Data Store Write2/1
  Subtract5/1 -> Data Store Write3/1
  SwitchPackRangeOffset8/1 -> Add3/2
  SwitchPackRangeOffset27/1 -> Subtract13/2
  SwitchPackRangeOffset24/1 -> Subtract15/2
  Subtract4/1 -> Data Store Write4/1
  SwitchPackRangeOffset9/1 -> Add4/2
  SwitchPackRangeOffset2/1 -> Add6/2
  Constant3/1 -> Subtract1/1, Add6/1, Subtract6/1, Subtract2/1, Add2/1, Add1/1
  Add6/1 -> Data Store Write11/1
  Subtract6/1 -> Data Store Write6/1
  Add2/1 -> Data Store Write10/1
  SwitchPackRangeOffset5/1 -> Add1/2
  SwitchPackRangeOffset6/1 -> Subtract3/2
  Subtract3/1 -> Data Store Write5/1
  SwitchPackRangeOffset4/1 -> Subtract2/2
  SwitchPackRangeOffset3/1 -> Subtract1/2
  SwitchPackRangeOffset1/1 -> Subtract6/2
  SwitchPackRangeOffset12/1 -> Add2/2
  Subtract1/1 -> Data Store Write9/1
  Add1/1 -> Data Store Write8/1
  Subtract8/1 -> Data Store Write16/1
  Add9/1 -> Data Store Write14/1
  SwitchPackRangeOffset10/1 -> Subtract9/2
  SwitchPackRangeOffset13/1 -> Add8/2
  Add8/1 -> Data Store Write13/1
  Subtract7/1 -> Data Store Write12/1
  Add7/1 -> Data Store Write17/1
  SwitchPackRangeOffset17/1 -> Add7/2
  SwitchPackRangeOffset14/1 -> Add9/2
  SwitchPackRangeOffset16/1 -> Subtract8/2
  SwitchPackRangeOffset15/1 -> Subtract7/2
  Constant5/1 -> Subtract7/1, Add8/1, Add9/1, Subtract9/1, Subtract8/1, Add7/1
  Subtract9/1 -> Data Store Write15/1
  SwitchPackRangeOffset18/1 -> Subtract10/2
  Subtract11/1 -> Data Store Write20/1
  Constant1/1 -> Add/1, Add10/1, Subtract10/1, Add11/1, Subtract11/1, Subtract/1
  SwitchPackRangeOffset/1 -> Subtract/2
  Subtract10/1 -> Data Store Write19/1
  SwitchPackRangeOffset19/1 -> Add/2
  Subtract/1 -> Data Store Write18/1
  SwitchPackRangeOffset22/1 -> Add11/2
  Add/1 -> Data Store Write23/1
  Add11/1 -> Data Store Write21/1
  SwitchPackRangeOffset21/1 -> Subtract11/2
  Add10/1 -> Data Store Write22/1
  SwitchPackRangeOffset20/1 -> Add10/2

== system amplifierboard/Motor_Control/Motor_Control/Chart/SendSPI ==
  DriverNo : Inport  OutDataTypeStr=uint8  PortDimensions=1
  SPICommand : Inport  Port=2  OutDataTypeStr=uint8  PortDimensions=[1 2]
  f : TriggerPort  TriggerType=function-call  VariantControl=(inherit)
      settings: CopyFcn=Stateflow.SLINSF.SimulinkMan.removeBlockPreDeleteFcn  PreDeleteFcn=Stateflow.SLINSF.SimulinkMan.unsafePredeleteFcn
  Merge : Merge  InitialOutput=0
  SPICommand1 : InportShadow  Port=2  OutDataTypeStr=uint8  PortDimensions=[1 2]
  Switch Case : SwitchCase  CaseConditions={1,2}  ShowDefaultCase=off
  Switch Case Action Subsystem : Subsystem  TreatAsAtomicUnit=on
  Switch Case Action Subsystem1 : Subsystem  TreatAsAtomicUnit=on
  StatusOut : Outport
  wires:
  DriverNo/1 -> Switch Case/1
  SPICommand/1 -> Switch Case Action Subsystem/1(SPI_Command1)
  Switch Case/1 -> Switch Case Action Subsystem/Action
  Switch Case Action Subsystem/1(Status_Out1) -> Merge/1
  Switch Case Action Subsystem1/1(Status_Out2) -> Merge/2
  SPICommand1/1 -> Switch Case Action Subsystem1/1(SPI_Command2)
  Switch Case/2 -> Switch Case Action Subsystem1/Action
  Merge/1 -> StatusOut/1

== system amplifierboard/CAN_Pack_And_Send/PsngrWndwCntDetect/SwtchPosDetect/FR_Dwn_CntDetect ==
  In1 : Inport
  Data Store Read31 : DataStoreRead  DataStoreName=FR_WindSw_Dwn_Cnts_Low
  Data Store Read32 : DataStoreRead  DataStoreName=FR_WindSw_Dwn_Cnts_Hi
  Logical Operator1 : Logic  AllPortsSameDT=off  OutDataTypeStr=boolean
  Relational Operator1 : RelationalOperator  Operator=<=  OutDataTypeStr=boolean  RndMeth=Simplest
  Relational Operator3 : RelationalOperator  OutDataTypeStr=boolean  RndMeth=Simplest
  Out1 : Outport
  wires:
  Data Store Read31/1 -> Relational Operator3/2
  In1/1 -> Relational Operator1/1, Relational Operator3/1  "In"
  Logical Operator1/1 -> Out1/1  "Out"
  Relational Operator3/1 -> Logical Operator1/2
  Data Store Read32/1 -> Relational Operator1/2
  Relational Operator1/1 -> Logical Operator1/1

== system amplifierboard/CAN_Pack_And_Send/PsngrWndwCntDetect/SwtchPosDetect/FR_ExpDwn_CntDetect ==
  In : Inport
  Data Store Read24 : DataStoreRead  DataStoreName=FR_WindSw_ExpDwn_Cnts_Low
  Data Store Read30 : DataStoreRead  DataStoreName=FR_WindSw_ExpDwn_Cnts_Hi
  Logical Operator : Logic  AllPortsSameDT=off  OutDataTypeStr=boolean
  Relational Operator : RelationalOperator  Operator=<=  OutDataTypeStr=boolean  RndMeth=Simplest
  Relational Operator2 : RelationalOperator  OutDataTypeStr=boolean  RndMeth=Simplest
  Out : Outport
  wires:
  In/1 -> Relational Operator/1, Relational Operator2/1  "In"
  Logical Operator/1 -> Out/1  "Out"
  Relational Operator2/1 -> Logical Operator/2
  Relational Operator/1 -> Logical Operator/1
  Data Store Read24/1 -> Relational Operator2/2
  Data Store Read30/1 -> Relational Operator/2

== system amplifierboard/CAN_Pack_And_Send/PsngrWndwCntDetect/SwtchPosDetect/FR_ExpUp_CntDetect ==
  In2 : Inport
  Data Store Read33 : DataStoreRead  DataStoreName=FR_WindSw_ExpUp_Cnts_Low
  Data Store Read34 : DataStoreRead  DataStoreName=FR_WindSw_ExpUp_Cnts_Hi
  Logical Operator2 : Logic  AllPortsSameDT=off  OutDataTypeStr=boolean
  Relational Operator4 : RelationalOperator  Operator=<=  OutDataTypeStr=boolean  RndMeth=Simplest
  Relational Operator5 : RelationalOperator  OutDataTypeStr=boolean  RndMeth=Simplest
  AutoRaiseCnt : Outport
  wires:
  Data Store Read33/1 -> Relational Operator5/2
  In2/1 -> Relational Operator4/1, Relational Operator5/1  "In"
  Logical Operator2/1 -> AutoRaiseCnt/1  "Out"
  Relational Operator5/1 -> Logical Operator2/2
  Data Store Read34/1 -> Relational Operator4/2
  Relational Operator4/1 -> Logical Operator2/1

== system amplifierboard/CAN_Pack_And_Send/PsngrWndwCntDetect/SwtchPosDetect/FR_NrmOpen_CntDetect ==
  In4 : Inport
  Data Store Read37 : DataStoreRead  DataStoreName=FR_WindSw_NrmOpen_Cnts_Low
  Data Store Read38 : DataStoreRead  DataStoreName=FR_WindSw_NrmOpen_Cnts_Hi
  Logical Operator4 : Logic  AllPortsSameDT=off  OutDataTypeStr=boolean
  Relational Operator8 : RelationalOperator  Operator=<=  OutDataTypeStr=boolean  RndMeth=Simplest
  Relational Operator9 : RelationalOperator  OutDataTypeStr=boolean  RndMeth=Simplest
  HoldCnt : Outport
  wires:
  Relational Operator8/1 -> Logical Operator4/1
  Data Store Read37/1 -> Relational Operator9/2
  Relational Operator9/1 -> Logical Operator4/2
  Data Store Read38/1 -> Relational Operator8/2
  In4/1 -> Relational Operator8/1, Relational Operator9/1  "In"
  Logical Operator4/1 -> HoldCnt/1  "Out"

== system amplifierboard/CAN_Pack_And_Send/PsngrWndwCntDetect/SwtchPosDetect/FR_Up_CntDetect ==
  In3 : Inport
  Data Store Read35 : DataStoreRead  DataStoreName=FR_WindSw_Up_Cnts_Low
  Data Store Read36 : DataStoreRead  DataStoreName=FR_WindSw_Up_Cnts_Hi
  Logical Operator3 : Logic  AllPortsSameDT=off  OutDataTypeStr=boolean
  Relational Operator6 : RelationalOperator  Operator=<=  OutDataTypeStr=boolean  RndMeth=Simplest
  Relational Operator7 : RelationalOperator  OutDataTypeStr=boolean  RndMeth=Simplest
  Out3 : Outport
  wires:
  Relational Operator6/1 -> Logical Operator3/1
  Data Store Read35/1 -> Relational Operator7/2
  Relational Operator7/1 -> Logical Operator3/2
  Data Store Read36/1 -> Relational Operator6/2
  In3/1 -> Relational Operator6/1, Relational Operator7/1  "In"
  Logical Operator3/1 -> Out3/1  "Out"

== system amplifierboard/CAN_Pack_And_Send/PsngrWndwCntDetect/SwtchPosDetect/SwitchPosDetect ==
  ManRaiseCnt : Inport
  ManLowerCnt : Inport  Port=2
  AutoRaiseCnt : Inport  Port=3
  AutoLowerCnt : Inport  Port=4
  HoldCnt : Inport  Port=5
  SwitchCount : Inport  Port=6
  AutoLowerVal : Constant  Value=AutoLowerVal
  AutoRaiseVal : Constant  Value=AutoRaiseVal
  HoldVal : Constant  Value=HoldVal
  ManualLowerVal : Constant  Value=ManualLowerVal
  ManualRaiseVal : Constant  Value=ManualRaiseVal
  Switch{,1..4} (5 alike) : Switch  Criteria=u2 ~= 0
  AvgCount : Outport
  wires:
  SwitchCount/1 -> Switch4/3  "SwitchCount"
  Switch4/1 -> Switch3/3
  HoldCnt/1 -> Switch4/2  "HoldCnt"
  ManLowerCnt/1 -> Switch1/2  "ManLowerCnt"
  AutoLowerCnt/1 -> Switch3/2  "AutoLowerCnt"
  Switch/1 -> AvgCount/1  "AvgCount"
  ManRaiseCnt/1 -> Switch/2  "ManRaiseCnt"
  ManualRaiseVal/1 -> Switch/1
  HoldVal/1 -> Switch4/1
  ManualLowerVal/1 -> Switch1/1
  AutoLowerVal/1 -> Switch3/1
  AutoRaiseVal/1 -> Switch2/1
  Switch3/1 -> Switch2/3
  Switch2/1 -> Switch1/3
  Switch1/1 -> Switch/3
  AutoRaiseCnt/1 -> Switch2/2  "AutoRaiseCnt"

== system amplifierboard/CAN_Pack_And_Send/RLWndwCntDetect/SwtchPosDetect/RL_Dwn_CntDetect ==
  In11 : Inport
  Data Store Read14 : DataStoreRead  DataStoreName=RL_WindSw_Dwn_Cnts_Low
  Data Store Read15 : DataStoreRead  DataStoreName=RL_WindSw_Dwn_Cnts_Hi
  Logical Operator11 : Logic  AllPortsSameDT=off  OutDataTypeStr=boolean
  Relational Operator21 : RelationalOperator  Operator=<=  OutDataTypeStr=boolean  RndMeth=Simplest
  Relational Operator23 : RelationalOperator  OutDataTypeStr=boolean  RndMeth=Simplest
  ManLowerCnt : Outport
  wires:
  In11/1 -> Relational Operator21/1, Relational Operator23/1  "In"
  Data Store Read14/1 -> Relational Operator23/2
  Data Store Read15/1 -> Relational Operator21/2
  Relational Operator23/1 -> Logical Operator11/2
  Logical Operator11/1 -> ManLowerCnt/1  "Out"
  Relational Operator21/1 -> Logical Operator11/1

== system amplifierboard/CAN_Pack_And_Send/RLWndwCntDetect/SwtchPosDetect/RL_ExpDwn_CntDetect ==
  In10 : Inport
  Data Store Read11 : DataStoreRead  DataStoreName=RL_WindSw_ExpDwn_Cnts_Low
  Data Store Read13 : DataStoreRead  DataStoreName=RL_WindSw_ExpDwn_Cnts_Hi
  Logical Operator10 : Logic  AllPortsSameDT=off  OutDataTypeStr=boolean
  Relational Operator20 : RelationalOperator  Operator=<=  OutDataTypeStr=boolean  RndMeth=Simplest
  Relational Operator22 : RelationalOperator  OutDataTypeStr=boolean  RndMeth=Simplest
  AutoLowerCnt : Outport
  wires:
  In10/1 -> Relational Operator20/1, Relational Operator22/1  "In"
  Logical Operator10/1 -> AutoLowerCnt/1  "Out"
  Relational Operator22/1 -> Logical Operator10/2
  Data Store Read11/1 -> Relational Operator22/2
  Data Store Read13/1 -> Relational Operator20/2
  Relational Operator20/1 -> Logical Operator10/1

== system amplifierboard/CAN_Pack_And_Send/RLWndwCntDetect/SwtchPosDetect/RL_ExpUp_CntDetect ==
  In12 : Inport
  Data Store Read16 : DataStoreRead  DataStoreName=RL_WindSw_ExpUp_Cnts_Low
  Data Store Read17 : DataStoreRead  DataStoreName=RL_WindSw_ExpUp_Cnts_Hi
  Logical Operator12 : Logic  AllPortsSameDT=off  OutDataTypeStr=boolean
  Relational Operator24 : RelationalOperator  Operator=<=  OutDataTypeStr=boolean  RndMeth=Simplest
  Relational Operator25 : RelationalOperator  OutDataTypeStr=boolean  RndMeth=Simplest
  Out12 : Outport
  wires:
  Data Store Read16/1 -> Relational Operator25/2
  Data Store Read17/1 -> Relational Operator24/2
  Relational Operator25/1 -> Logical Operator12/2
  Relational Operator24/1 -> Logical Operator12/1
  In12/1 -> Relational Operator24/1, Relational Operator25/1  "In"
  Logical Operator12/1 -> Out12/1  "Out"

== system amplifierboard/CAN_Pack_And_Send/RLWndwCntDetect/SwtchPosDetect/RL_NrmOpen_CntDetect ==
  In14 : Inport
  Data Store Read12 : DataStoreRead  DataStoreName=RL_WindSw_NrmOpen_Cnts_Hi
  Data Store Read20 : DataStoreRead  DataStoreName=RL_WindSw_NrmOpen_Cnts_Low
  Logical Operator14 : Logic  AllPortsSameDT=off  OutDataTypeStr=boolean
  Relational Operator28 : RelationalOperator  Operator=<=  OutDataTypeStr=boolean  RndMeth=Simplest
  Relational Operator29 : RelationalOperator  OutDataTypeStr=boolean  RndMeth=Simplest
  HoldCnt : Outport
  wires:
  Relational Operator28/1 -> Logical Operator14/1
  Data Store Read20/1 -> Relational Operator29/2
  Relational Operator29/1 -> Logical Operator14/2
  Data Store Read12/1 -> Relational Operator28/2
  Logical Operator14/1 -> HoldCnt/1  "Out"
  In14/1 -> Relational Operator28/1, Relational Operator29/1  "In"

== system amplifierboard/CAN_Pack_And_Send/RLWndwCntDetect/SwtchPosDetect/RL_Up_CntDetect ==
  In13 : Inport
  Data Store Read18 : DataStoreRead  DataStoreName=RL_WindSw_Up_Cnts_Low
  Data Store Read19 : DataStoreRead  DataStoreName=RL_WindSw_Up_Cnts_Hi
  Logical Operator13 : Logic  AllPortsSameDT=off  OutDataTypeStr=boolean
  Relational Operator26 : RelationalOperator  Operator=<=  OutDataTypeStr=boolean  RndMeth=Simplest
  Relational Operator27 : RelationalOperator  OutDataTypeStr=boolean  RndMeth=Simplest
  Out13 : Outport
  wires:
  Relational Operator27/1 -> Logical Operator13/2
  Data Store Read19/1 -> Relational Operator26/2
  Data Store Read18/1 -> Relational Operator27/2
  Relational Operator26/1 -> Logical Operator13/1
  Logical Operator13/1 -> Out13/1  "Out"
  In13/1 -> Relational Operator26/1, Relational Operator27/1  "In"

== system amplifierboard/CAN_Pack_And_Send/RLWndwCntDetect/SwtchPosDetect/SwitchPosDetect2 ==
  ManRaiseCnt : Inport
  ManLowerCnt : Inport  Port=2
  AutoRaiseCnt : Inport  Port=3
  AutoLowerCnt : Inport  Port=4
  HoldCnt : Inport  Port=5
  SwitchCount : Inport  Port=6
  AutoLowerVal : Constant  Value=AutoLowerVal
  AutoRaiseVal : Constant  Value=AutoRaiseVal
  HoldVal : Constant  Value=HoldVal
  ManualLowerVal : Constant  Value=ManualLowerVal
  ManualRaiseVal : Constant  Value=ManualRaiseVal
  Switch{,1..4} (5 alike) : Switch  Criteria=u2 ~= 0
  AvgCount : Outport
  wires:
  SwitchCount/1 -> Switch4/3  "SwitchCount"
  Switch4/1 -> Switch3/3
  HoldCnt/1 -> Switch4/2  "HoldCnt"
  ManLowerCnt/1 -> Switch1/2  "ManLowerCnt"
  AutoLowerCnt/1 -> Switch3/2  "AutoLowerCnt"
  Switch/1 -> AvgCount/1  "AvgCount"
  ManRaiseCnt/1 -> Switch/2  "ManRaiseCnt"
  ManualRaiseVal/1 -> Switch/1
  HoldVal/1 -> Switch4/1
  ManualLowerVal/1 -> Switch1/1
  AutoLowerVal/1 -> Switch3/1
  AutoRaiseVal/1 -> Switch2/1
  Switch3/1 -> Switch2/3
  Switch2/1 -> Switch1/3
  Switch1/1 -> Switch/3
  AutoRaiseCnt/1 -> Switch2/2  "AutoRaiseCnt"
